simulink model "controller_position_down"  (R2021a)
settings: Solver=FixedStepAuto  StartTime=0.0  StopTime=10.0  FixedStep=0.002  RelTol=1e-3
undefined symbols (not defined in the file): G_PD_OL_DENOM, G_PD_OL_NUM, K_dp
settings Model: Creator=francois  LastModifiedBy=esl
settings SolverCC: AlgebraicLoopSolver=TrustRegion
settings DebuggingCC: SFMachineParentedDataDiag=warning

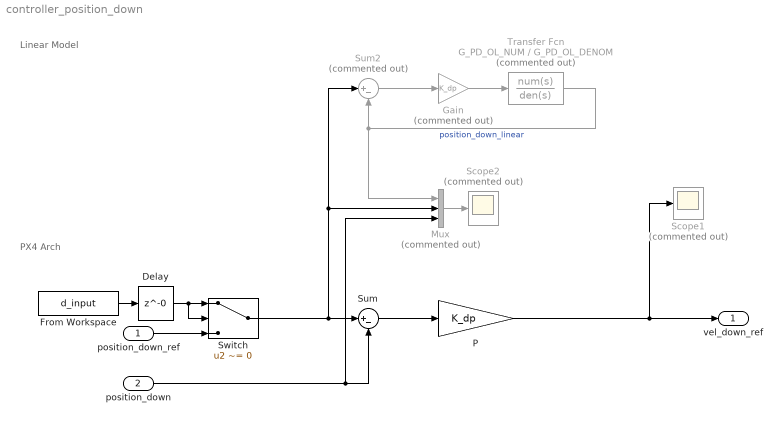
== system controller_position_down ==
  note: PX4 Arch
  note: Linear Model
  position_down_ref : Inport
  position_down : Inport  Port=2
  Delay : Delay  DelayLength=0
  From Workspace : FromWorkspace  VariableName=d_input
  Gain : Gain  Commented=on  Gain=K_dp
  Mux : Mux  Commented=on  Inputs=3
  P : Gain  Gain=K_dp
  Scope1 : Scope  Commented=on
  Scope2 : Scope  Commented=on
  Sum : Sum  Inputs=|+-
  Sum2 : Sum  Commented=on  Inputs=|+-
  Switch : Switch  Criteria=u2 ~= 0
  Transfer Fcn : TransferFcn  Commented=on  Numerator=G_PD_OL_NUM  Denominator=G_PD_OL_DENOM
  vel_down_ref : Outport  VectorParamsAs1DForOutWhenUnconnected=off
  wires:
  From Workspace/1 -> Delay/1
  Sum2/1 -> Gain/1
  Gain/1 -> Transfer Fcn/1
  P/1 -> vel_down_ref/1, Scope1/1
  Switch/1 -> Sum/1, Mux/2, Sum2/1
  position_down_ref/1 -> Switch/3
  Transfer Fcn/1 -> Mux/1, Sum2/2  "position_down_linear"
  Sum/1 -> P/1
  Delay/1 -> Switch/2, Switch/1
  position_down/1 -> Mux/3, Sum/2
  Mux/1 -> Scope2/1
